simulink model "xhand_sphere_tube_r2021b"  (R2021b)
settings: Solver=VariableStepAuto  StartTime=0.0  StopTime=20  RelTol=1e-3
InitFcn:
  | radium=0.045
undefined symbols (not defined in the file): X, Y, Z
libraries: sm_lib x120, nesl_utility x26, Contact_Forces_Lib x21
(part 2 of 4)

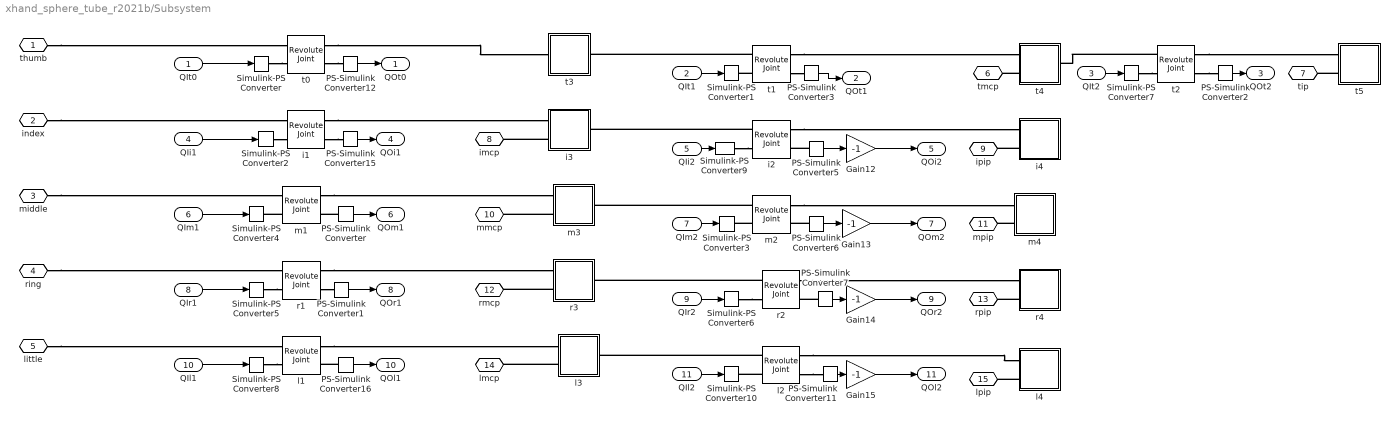
== system xhand_sphere_tube_r2021b/Subsystem ==
  QIt0 : Inport
  QIt1 : Inport  Port=2
  QIt2 : Inport  Port=3
  QIi1 : Inport  Port=4
  QIi2 : Inport  Port=5
  QIm1 : Inport  Port=6
  QIm2 : Inport  Port=7
  QIr1 : Inport  Port=8
  QIr2 : Inport  Port=9
  QIl1 : Inport  Port=10
  QIl2 : Inport  Port=11
  Gain{12..15} (4 alike) : Gain  Gain=-1
  PS-Simulink Converter{,1..3,5..7,11..12,15..16} (11 alike) : nesl_utility/PS-Simulink Converter  PhysicalDomain=network_engine_domain  SubClassName=ps_output  LeftPortType=input  RightPortType=output  PseudoPeriodic=off  Frequencies=[]  Unit=inherit  AffineConversion=off
      settings: SourceProductBaseCode=PW,SS
  Simulink-PS Converter{,1..10} (11 alike) : nesl_utility/Simulink-PS Converter  PhysicalDomain=network_engine_domain  SubClassName=ps_input  LeftPortType=input  RightPortType=output  PseudoPeriodic=off  Frequencies=[]  NoiseDistribution=none  NoiseParameters=[]  Unit=1  AffineConversion=off  FilteringAndDerivatives=filter  SimscapeFilterOrder=2  InputFilterTimeConstant=0.001  UdotUserProvided=0
      settings: SourceProductBaseCode=PW,SS
  i1 : sm_lib/Joints/Revolute Joint  JointMode=Normal  SenseConstraintForce=off  SenseConstraintForceX=off  SenseConstraintForceY=off  SenseConstraintForceZ=off  SenseConstraintTorque=off  SenseConstraintTorqueX=off  SenseConstraintTorqueY=off  SenseConstraintTorqueZ=off  SenseTotalForce=off  SenseTotalForceX=off  SenseTotalForceY=off  SenseTotalForceZ=off  SenseTotalTorque=off  SenseTotalTorqueX=off  SenseTotalTorqueY=off  SenseTotalTorqueZ=off  CompositeWrenchDir=FollowerOnBase  CompositeWrenchFrame=BaseFrame  EquilibriumPosition=0  EquilibriumPositionUnits=deg  SpringStiffness=0  SpringStiffnessUnits=N*m/deg  DampingCoefficient=0  DampingCoefficientUnits=m^2*kg/s/rad  TorqueActuationMode=ComputedTorque  MotionActuationMode=InputMotion  SensePosition=on  SenseVelocity=off  SenseAcceleration=off  SenseTorqueForce=off  SenseLowerLimitTorqueForce=off  SenseUpperLimitTorqueForce=off  LowerLimitSpecify=on  LowerLimitBound=-3.14  LowerLimitBoundUnits=rad  LowerLimitStiffness=1e4  LowerLimitStiffnessUnits=N*m/deg  LowerLimitDamping=10  LowerLimitDampingUnits=N*m/(deg/s)  LowerLimitTransitionRegionWidth=0.1  LowerLimitTransitionRegionWidthUnits=deg  UpperLimitSpecify=on  UpperLimitBound=3.14  UpperLimitBoundUnits=rad  UpperLimitStiffness=1e4  UpperLimitStiffnessUnits=N*m/deg  UpperLimitDamping=10  UpperLimitDampingUnits=N*m/(deg/s)  UpperLimitTransitionRegionWidth=0.1  UpperLimitTransitionRegionWidthUnits=deg  PositionTargetSpecify=off  PositionTargetPriority=High  PositionTargetValue=0  PositionTargetValueUnits=deg  VelocityTargetSpecify=off  VelocityTargetPriority=High  VelocityTargetValue=0  VelocityTargetValueUnits=deg/s
  i2 : sm_lib/Joints/Revolute Joint  JointMode=Normal  SenseConstraintForce=off  SenseConstraintForceX=off  SenseConstraintForceY=off  SenseConstraintForceZ=off  SenseConstraintTorque=off  SenseConstraintTorqueX=off  SenseConstraintTorqueY=off  SenseConstraintTorqueZ=off  SenseTotalForce=off  SenseTotalForceX=off  SenseTotalForceY=off  SenseTotalForceZ=off  SenseTotalTorque=off  SenseTotalTorqueX=off  SenseTotalTorqueY=off  SenseTotalTorqueZ=off  CompositeWrenchDir=FollowerOnBase  CompositeWrenchFrame=BaseFrame  EquilibriumPosition=0  EquilibriumPositionUnits=deg  SpringStiffness=0  SpringStiffnessUnits=N*m/deg  DampingCoefficient=0  DampingCoefficientUnits=m^2*kg/s/rad  TorqueActuationMode=ComputedTorque  MotionActuationMode=InputMotion  SensePosition=on  SenseVelocity=off  SenseAcceleration=off  SenseTorqueForce=off  SenseLowerLimitTorqueForce=off  SenseUpperLimitTorqueForce=off  LowerLimitSpecify=on  LowerLimitBound=-3.14  LowerLimitBoundUnits=rad  LowerLimitStiffness=1e4  LowerLimitStiffnessUnits=N*m/deg  LowerLimitDamping=10  LowerLimitDampingUnits=N*m/(deg/s)  LowerLimitTransitionRegionWidth=0.1  LowerLimitTransitionRegionWidthUnits=deg  UpperLimitSpecify=on  UpperLimitBound=3.14  UpperLimitBoundUnits=rad  UpperLimitStiffness=1e4  UpperLimitStiffnessUnits=N*m/deg  UpperLimitDamping=10  UpperLimitDampingUnits=N*m/(deg/s)  UpperLimitTransitionRegionWidth=0.1  UpperLimitTransitionRegionWidthUnits=deg  PositionTargetSpecify=off  PositionTargetPriority=High  PositionTargetValue=0  PositionTargetValueUnits=deg  VelocityTargetSpecify=off  VelocityTargetPriority=High  VelocityTargetValue=0  VelocityTargetValueUnits=deg/s
  i3 : Subsystem
  i4 : Subsystem
  l1 : sm_lib/Joints/Revolute Joint  JointMode=Normal  SenseConstraintForce=off  SenseConstraintForceX=off  SenseConstraintForceY=off  SenseConstraintForceZ=off  SenseConstraintTorque=off  SenseConstraintTorqueX=off  SenseConstraintTorqueY=off  SenseConstraintTorqueZ=off  SenseTotalForce=off  SenseTotalForceX=off  SenseTotalForceY=off  SenseTotalForceZ=off  SenseTotalTorque=off  SenseTotalTorqueX=off  SenseTotalTorqueY=off  SenseTotalTorqueZ=off  CompositeWrenchDir=FollowerOnBase  CompositeWrenchFrame=BaseFrame  EquilibriumPosition=0  EquilibriumPositionUnits=deg  SpringStiffness=0  SpringStiffnessUnits=N*m/deg  DampingCoefficient=0  DampingCoefficientUnits=m^2*kg/s/rad  TorqueActuationMode=ComputedTorque  MotionActuationMode=InputMotion  SensePosition=on  SenseVelocity=off  SenseAcceleration=off  SenseTorqueForce=off  SenseLowerLimitTorqueForce=off  SenseUpperLimitTorqueForce=off  LowerLimitSpecify=on  LowerLimitBound=-3.14  LowerLimitBoundUnits=rad  LowerLimitStiffness=1e4  LowerLimitStiffnessUnits=N*m/deg  LowerLimitDamping=10  LowerLimitDampingUnits=N*m/(deg/s)  LowerLimitTransitionRegionWidth=0.1  LowerLimitTransitionRegionWidthUnits=deg  UpperLimitSpecify=on  UpperLimitBound=3.14  UpperLimitBoundUnits=rad  UpperLimitStiffness=1e4  UpperLimitStiffnessUnits=N*m/deg  UpperLimitDamping=10  UpperLimitDampingUnits=N*m/(deg/s)  UpperLimitTransitionRegionWidth=0.1  UpperLimitTransitionRegionWidthUnits=deg  PositionTargetSpecify=off  PositionTargetPriority=High  PositionTargetValue=0  PositionTargetValueUnits=deg  VelocityTargetSpecify=off  VelocityTargetPriority=High  VelocityTargetValue=0  VelocityTargetValueUnits=deg/s
  l2 : sm_lib/Joints/Revolute Joint  JointMode=Normal  SenseConstraintForce=off  SenseConstraintForceX=off  SenseConstraintForceY=off  SenseConstraintForceZ=off  SenseConstraintTorque=off  SenseConstraintTorqueX=off  SenseConstraintTorqueY=off  SenseConstraintTorqueZ=off  SenseTotalForce=off  SenseTotalForceX=off  SenseTotalForceY=off  SenseTotalForceZ=off  SenseTotalTorque=off  SenseTotalTorqueX=off  SenseTotalTorqueY=off  SenseTotalTorqueZ=off  CompositeWrenchDir=FollowerOnBase  CompositeWrenchFrame=BaseFrame  EquilibriumPosition=0  EquilibriumPositionUnits=deg  SpringStiffness=0  SpringStiffnessUnits=N*m/deg  DampingCoefficient=0  DampingCoefficientUnits=m^2*kg/s/rad  TorqueActuationMode=ComputedTorque  MotionActuationMode=InputMotion  SensePosition=on  SenseVelocity=off  SenseAcceleration=off  SenseTorqueForce=off  SenseLowerLimitTorqueForce=off  SenseUpperLimitTorqueForce=off  LowerLimitSpecify=on  LowerLimitBound=-3.14  LowerLimitBoundUnits=rad  LowerLimitStiffness=1e4  LowerLimitStiffnessUnits=N*m/deg  LowerLimitDamping=10  LowerLimitDampingUnits=N*m/(deg/s)  LowerLimitTransitionRegionWidth=0.1  LowerLimitTransitionRegionWidthUnits=deg  UpperLimitSpecify=on  UpperLimitBound=3.14  UpperLimitBoundUnits=rad  UpperLimitStiffness=1e4  UpperLimitStiffnessUnits=N*m/deg  UpperLimitDamping=10  UpperLimitDampingUnits=N*m/(deg/s)  UpperLimitTransitionRegionWidth=0.1  UpperLimitTransitionRegionWidthUnits=deg  PositionTargetSpecify=off  PositionTargetPriority=High  PositionTargetValue=0  PositionTargetValueUnits=deg  VelocityTargetSpecify=off  VelocityTargetPriority=High  VelocityTargetValue=0  VelocityTargetValueUnits=deg/s
  l3 : Subsystem
  l4 : Subsystem
  m1 : sm_lib/Joints/Revolute Joint  JointMode=Normal  SenseConstraintForce=off  SenseConstraintForceX=off  SenseConstraintForceY=off  SenseConstraintForceZ=off  SenseConstraintTorque=off  SenseConstraintTorqueX=off  SenseConstraintTorqueY=off  SenseConstraintTorqueZ=off  SenseTotalForce=off  SenseTotalForceX=off  SenseTotalForceY=off  SenseTotalForceZ=off  SenseTotalTorque=off  SenseTotalTorqueX=off  SenseTotalTorqueY=off  SenseTotalTorqueZ=off  CompositeWrenchDir=FollowerOnBase  CompositeWrenchFrame=BaseFrame  EquilibriumPosition=0  EquilibriumPositionUnits=deg  SpringStiffness=0  SpringStiffnessUnits=N*m/deg  DampingCoefficient=0.000005  DampingCoefficientUnits=m^2*kg/s/rad  TorqueActuationMode=ComputedTorque  MotionActuationMode=InputMotion  SensePosition=on  SenseVelocity=off  SenseAcceleration=off  SenseTorqueForce=off  SenseLowerLimitTorqueForce=off  SenseUpperLimitTorqueForce=off  LowerLimitSpecify=on  LowerLimitBound=-3.14  LowerLimitBoundUnits=rad  LowerLimitStiffness=1e4  LowerLimitStiffnessUnits=N*m/deg  LowerLimitDamping=10  LowerLimitDampingUnits=N*m/(deg/s)  LowerLimitTransitionRegionWidth=0.1  LowerLimitTransitionRegionWidthUnits=deg  UpperLimitSpecify=on  UpperLimitBound=3.14  UpperLimitBoundUnits=rad  UpperLimitStiffness=1e4  UpperLimitStiffnessUnits=N*m/deg  UpperLimitDamping=10  UpperLimitDampingUnits=N*m/(deg/s)  UpperLimitTransitionRegionWidth=0.1  UpperLimitTransitionRegionWidthUnits=deg  PositionTargetSpecify=off  PositionTargetPriority=High  PositionTargetValue=0  PositionTargetValueUnits=deg  VelocityTargetSpecify=off  VelocityTargetPriority=High  VelocityTargetValue=0  VelocityTargetValueUnits=deg/s
  m2 : sm_lib/Joints/Revolute Joint  JointMode=Normal  SenseConstraintForce=off  SenseConstraintForceX=off  SenseConstraintForceY=off  SenseConstraintForceZ=off  SenseConstraintTorque=off  SenseConstraintTorqueX=off  SenseConstraintTorqueY=off  SenseConstraintTorqueZ=off  SenseTotalForce=off  SenseTotalForceX=off  SenseTotalForceY=off  SenseTotalForceZ=off  SenseTotalTorque=off  SenseTotalTorqueX=off  SenseTotalTorqueY=off  SenseTotalTorqueZ=off  CompositeWrenchDir=FollowerOnBase  CompositeWrenchFrame=BaseFrame  EquilibriumPosition=0  EquilibriumPositionUnits=deg  SpringStiffness=0  SpringStiffnessUnits=N*m/deg  DampingCoefficient=0  DampingCoefficientUnits=m^2*kg/s/rad  TorqueActuationMode=ComputedTorque  MotionActuationMode=InputMotion  SensePosition=on  SenseVelocity=off  SenseAcceleration=off  SenseTorqueForce=off  SenseLowerLimitTorqueForce=off  SenseUpperLimitTorqueForce=off  LowerLimitSpecify=on  LowerLimitBound=-3.14  LowerLimitBoundUnits=rad  LowerLimitStiffness=1e4  LowerLimitStiffnessUnits=N*m/deg  LowerLimitDamping=10  LowerLimitDampingUnits=N*m/(deg/s)  LowerLimitTransitionRegionWidth=0.1  LowerLimitTransitionRegionWidthUnits=deg  UpperLimitSpecify=on  UpperLimitBound=3.14  UpperLimitBoundUnits=rad  UpperLimitStiffness=1e4  UpperLimitStiffnessUnits=N*m/deg  UpperLimitDamping=10  UpperLimitDampingUnits=N*m/(deg/s)  UpperLimitTransitionRegionWidth=0.1  UpperLimitTransitionRegionWidthUnits=deg  PositionTargetSpecify=off  PositionTargetPriority=High  PositionTargetValue=0  PositionTargetValueUnits=deg  VelocityTargetSpecify=off  VelocityTargetPriority=High  VelocityTargetValue=0  VelocityTargetValueUnits=deg/s
  m3 : Subsystem
  m4 : Subsystem
  r1 : sm_lib/Joints/Revolute Joint  JointMode=Normal  SenseConstraintForce=off  SenseConstraintForceX=off  SenseConstraintForceY=off  SenseConstraintForceZ=off  SenseConstraintTorque=off  SenseConstraintTorqueX=off  SenseConstraintTorqueY=off  SenseConstraintTorqueZ=off  SenseTotalForce=off  SenseTotalForceX=off  SenseTotalForceY=off  SenseTotalForceZ=off  SenseTotalTorque=off  SenseTotalTorqueX=off  SenseTotalTorqueY=off  SenseTotalTorqueZ=off  CompositeWrenchDir=FollowerOnBase  CompositeWrenchFrame=BaseFrame  EquilibriumPosition=0  EquilibriumPositionUnits=deg  SpringStiffness=0  SpringStiffnessUnits=N*m/deg  DampingCoefficient=0.00005  DampingCoefficientUnits=m^2*kg/s/rad  TorqueActuationMode=ComputedTorque  MotionActuationMode=InputMotion  SensePosition=on  SenseVelocity=off  SenseAcceleration=off  SenseTorqueForce=off  SenseLowerLimitTorqueForce=off  SenseUpperLimitTorqueForce=off  LowerLimitSpecify=on  LowerLimitBound=-3.14  LowerLimitBoundUnits=rad  LowerLimitStiffness=1e4  LowerLimitStiffnessUnits=N*m/deg  LowerLimitDamping=10  LowerLimitDampingUnits=N*m/(deg/s)  LowerLimitTransitionRegionWidth=0.1  LowerLimitTransitionRegionWidthUnits=deg  UpperLimitSpecify=on  UpperLimitBound=3.14  UpperLimitBoundUnits=rad  UpperLimitStiffness=1e4  UpperLimitStiffnessUnits=N*m/deg  UpperLimitDamping=10  UpperLimitDampingUnits=N*m/(deg/s)  UpperLimitTransitionRegionWidth=0.1  UpperLimitTransitionRegionWidthUnits=deg  PositionTargetSpecify=off  PositionTargetPriority=High  PositionTargetValue=0  PositionTargetValueUnits=deg  VelocityTargetSpecify=off  VelocityTargetPriority=High  VelocityTargetValue=0  VelocityTargetValueUnits=deg/s
  r2 : sm_lib/Joints/Revolute Joint  JointMode=Normal  SenseConstraintForce=off  SenseConstraintForceX=off  SenseConstraintForceY=off  SenseConstraintForceZ=off  SenseConstraintTorque=off  SenseConstraintTorqueX=off  SenseConstraintTorqueY=off  SenseConstraintTorqueZ=off  SenseTotalForce=off  SenseTotalForceX=off  SenseTotalForceY=off  SenseTotalForceZ=off  SenseTotalTorque=off  SenseTotalTorqueX=off  SenseTotalTorqueY=off  SenseTotalTorqueZ=off  CompositeWrenchDir=FollowerOnBase  CompositeWrenchFrame=BaseFrame  EquilibriumPosition=0  EquilibriumPositionUnits=deg  SpringStiffness=0  SpringStiffnessUnits=N*m/deg  DampingCoefficient=0  DampingCoefficientUnits=m^2*kg/s/rad  TorqueActuationMode=ComputedTorque  MotionActuationMode=InputMotion  SensePosition=on  SenseVelocity=off  SenseAcceleration=off  SenseTorqueForce=off  SenseLowerLimitTorqueForce=off  SenseUpperLimitTorqueForce=off  LowerLimitSpecify=on  LowerLimitBound=-3.14  LowerLimitBoundUnits=rad  LowerLimitStiffness=1e4  LowerLimitStiffnessUnits=N*m/deg  LowerLimitDamping=10  LowerLimitDampingUnits=N*m/(deg/s)  LowerLimitTransitionRegionWidth=0.1  LowerLimitTransitionRegionWidthUnits=deg  UpperLimitSpecify=on  UpperLimitBound=3.14  UpperLimitBoundUnits=rad  UpperLimitStiffness=1e4  UpperLimitStiffnessUnits=N*m/deg  UpperLimitDamping=10  UpperLimitDampingUnits=N*m/(deg/s)  UpperLimitTransitionRegionWidth=0.1  UpperLimitTransitionRegionWidthUnits=deg  PositionTargetSpecify=off  PositionTargetPriority=High  PositionTargetValue=0  PositionTargetValueUnits=deg  VelocityTargetSpecify=off  VelocityTargetPriority=High  VelocityTargetValue=0  VelocityTargetValueUnits=deg/s
  r3 : Subsystem
  r4 : Subsystem
  t0 : sm_lib/Joints/Revolute Joint  JointMode=Normal  SenseConstraintForce=off  SenseConstraintForceX=off  SenseConstraintForceY=off  SenseConstraintForceZ=off  SenseConstraintTorque=off  SenseConstraintTorqueX=off  SenseConstraintTorqueY=off  SenseConstraintTorqueZ=off  SenseTotalForce=off  SenseTotalForceX=off  SenseTotalForceY=off  SenseTotalForceZ=off  SenseTotalTorque=off  SenseTotalTorqueX=off  SenseTotalTorqueY=off  SenseTotalTorqueZ=off  CompositeWrenchDir=FollowerOnBase  CompositeWrenchFrame=BaseFrame  EquilibriumPosition=0  EquilibriumPositionUnits=deg  SpringStiffness=0  SpringStiffnessUnits=N*m/deg  DampingCoefficient=0  DampingCoefficientUnits=m^2*kg/s/rad  TorqueActuationMode=ComputedTorque  MotionActuationMode=InputMotion  SensePosition=on  SenseVelocity=off  SenseAcceleration=off  SenseTorqueForce=off  SenseLowerLimitTorqueForce=off  SenseUpperLimitTorqueForce=off  LowerLimitSpecify=on  LowerLimitBound=-3.14  LowerLimitBoundUnits=rad  LowerLimitStiffness=1e4  LowerLimitStiffnessUnits=N*m/deg  LowerLimitDamping=10  LowerLimitDampingUnits=N*m/(deg/s)  LowerLimitTransitionRegionWidth=0.1  LowerLimitTransitionRegionWidthUnits=deg  UpperLimitSpecify=on  UpperLimitBound=3.14  UpperLimitBoundUnits=rad  UpperLimitStiffness=1e4  UpperLimitStiffnessUnits=N*m/deg  UpperLimitDamping=10  UpperLimitDampingUnits=N*m/(deg/s)  UpperLimitTransitionRegionWidth=0.1  UpperLimitTransitionRegionWidthUnits=deg  PositionTargetSpecify=off  PositionTargetPriority=High  PositionTargetValue=0  PositionTargetValueUnits=deg  VelocityTargetSpecify=off  VelocityTargetPriority=High  VelocityTargetValue=0  VelocityTargetValueUnits=deg/s
  t1 : sm_lib/Joints/Revolute Joint  JointMode=Normal  SenseConstraintForce=off  SenseConstraintForceX=off  SenseConstraintForceY=off  SenseConstraintForceZ=off  SenseConstraintTorque=off  SenseConstraintTorqueX=off  SenseConstraintTorqueY=off  SenseConstraintTorqueZ=off  SenseTotalForce=off  SenseTotalForceX=off  SenseTotalForceY=off  SenseTotalForceZ=off  SenseTotalTorque=off  SenseTotalTorqueX=off  SenseTotalTorqueY=off  SenseTotalTorqueZ=off  CompositeWrenchDir=FollowerOnBase  CompositeWrenchFrame=BaseFrame  EquilibriumPosition=0  EquilibriumPositionUnits=deg  SpringStiffness=0  SpringStiffnessUnits=N*m/deg  DampingCoefficient=0  DampingCoefficientUnits=m^2*kg/s/rad  TorqueActuationMode=ComputedTorque  MotionActuationMode=InputMotion  SensePosition=on  SenseVelocity=off  SenseAcceleration=off  SenseTorqueForce=off  SenseLowerLimitTorqueForce=off  SenseUpperLimitTorqueForce=off  LowerLimitSpecify=on  LowerLimitBound=-3.14  LowerLimitBoundUnits=rad  LowerLimitStiffness=1e4  LowerLimitStiffnessUnits=N*m/deg  LowerLimitDamping=10  LowerLimitDampingUnits=N*m/(deg/s)  LowerLimitTransitionRegionWidth=0.1  LowerLimitTransitionRegionWidthUnits=deg  UpperLimitSpecify=on  UpperLimitBound=3.14  UpperLimitBoundUnits=rad  UpperLimitStiffness=1e4  UpperLimitStiffnessUnits=N*m/deg  UpperLimitDamping=10  UpperLimitDampingUnits=N*m/(deg/s)  UpperLimitTransitionRegionWidth=0.1  UpperLimitTransitionRegionWidthUnits=deg  PositionTargetSpecify=off  PositionTargetPriority=High  PositionTargetValue=0  PositionTargetValueUnits=deg  VelocityTargetSpecify=off  VelocityTargetPriority=High  VelocityTargetValue=0  VelocityTargetValueUnits=deg/s
  t2 : sm_lib/Joints/Revolute Joint  JointMode=Normal  SenseConstraintForce=off  SenseConstraintForceX=off  SenseConstraintForceY=off  SenseConstraintForceZ=off  SenseConstraintTorque=off  SenseConstraintTorqueX=off  SenseConstraintTorqueY=off  SenseConstraintTorqueZ=off  SenseTotalForce=off  SenseTotalForceX=off  SenseTotalForceY=off  SenseTotalForceZ=off  SenseTotalTorque=off  SenseTotalTorqueX=off  SenseTotalTorqueY=off  SenseTotalTorqueZ=off  CompositeWrenchDir=FollowerOnBase  CompositeWrenchFrame=BaseFrame  EquilibriumPosition=0  EquilibriumPositionUnits=deg  SpringStiffness=0  SpringStiffnessUnits=N*m/deg  DampingCoefficient=0  DampingCoefficientUnits=m^2*kg/s/rad  TorqueActuationMode=ComputedTorque  MotionActuationMode=InputMotion  SensePosition=on  SenseVelocity=off  SenseAcceleration=off  SenseTorqueForce=off  SenseLowerLimitTorqueForce=off  SenseUpperLimitTorqueForce=off  LowerLimitSpecify=on  LowerLimitBound=-3.14  LowerLimitBoundUnits=rad  LowerLimitStiffness=1e4  LowerLimitStiffnessUnits=N*m/deg  LowerLimitDamping=10  LowerLimitDampingUnits=N*m/(deg/s)  LowerLimitTransitionRegionWidth=0.1  LowerLimitTransitionRegionWidthUnits=deg  UpperLimitSpecify=on  UpperLimitBound=3.14  UpperLimitBoundUnits=rad  UpperLimitStiffness=1e4  UpperLimitStiffnessUnits=N*m/deg  UpperLimitDamping=10  UpperLimitDampingUnits=N*m/(deg/s)  UpperLimitTransitionRegionWidth=0.1  UpperLimitTransitionRegionWidthUnits=deg  PositionTargetSpecify=off  PositionTargetPriority=High  PositionTargetValue=0  PositionTargetValueUnits=deg  VelocityTargetSpecify=off  VelocityTargetPriority=High  VelocityTargetValue=0  VelocityTargetValueUnits=deg/s
  t3 : Subsystem
  t4 : Subsystem
  t5 : Subsystem
  thumb : PMIOPort  Side=Left
  index : PMIOPort  Port=2  Side=Left
  middle : PMIOPort  Port=3  Side=Left
  ring : PMIOPort  Port=4  Side=Left
  little : PMIOPort  Port=5  Side=Left
  tmcp : PMIOPort  Port=6  Side=Left
  tip : PMIOPort  Port=7  Side=Left
  imcp : PMIOPort  Port=8  Side=Left
  ipip : PMIOPort  Port=9  Side=Left
  mmcp : PMIOPort  Port=10  Side=Left
  mpip : PMIOPort  Port=11  Side=Left
  rmcp : PMIOPort  Port=12  Side=Left
  rpip : PMIOPort  Port=13  Side=Left
  lmcp : PMIOPort  Port=14  Side=Left
  lpip : PMIOPort  Port=15  Side=Left
  QOt0 : Outport
  QOt1 : Outport  Port=2
  QOt2 : Outport  Port=3
  QOi1 : Outport  Port=4
  QOi2 : Outport  Port=5
  QOm1 : Outport  Port=6
  QOm2 : Outport  Port=7
  QOr1 : Outport  Port=8
  QOr2 : Outport  Port=9
  QOl1 : Outport  Port=10
  QOl2 : Outport  Port=11
  wires:
  Gain13/1 -> QOm2/1
  PS-Simulink Converter5/1 -> Gain12/1
  QIm2/1 -> Simulink-PS Converter3/1
  QIt1/1 -> Simulink-PS Converter1/1
  PS-Simulink Converter11/1 -> Gain15/1
  PS-Simulink Converter6/1 -> Gain13/1
  PS-Simulink Converter2/1 -> QOt2/1
  Gain14/1 -> QOr2/1
  PS-Simulink Converter7/1 -> Gain14/1
  Gain12/1 -> QOi2/1
  PS-Simulink Converter12/1 -> QOt0/1
  QIr1/1 -> Simulink-PS Converter5/1
  PS-Simulink Converter/1 -> QOm1/1
  PS-Simulink Converter1/1 -> QOr1/1
  Gain15/1 -> QOl2/1
  PS-Simulink Converter16/1 -> QOl1/1
  PS-Simulink Converter3/1 -> QOt1/1
  QIi2/1 -> Simulink-PS Converter9/1
  QIr2/1 -> Simulink-PS Converter6/1
  QIl2/1 -> Simulink-PS Converter10/1
  QIi1/1 -> Simulink-PS Converter2/1
  QIt0/1 -> Simulink-PS Converter/1
  QIl1/1 -> Simulink-PS Converter8/1
  QIm1/1 -> Simulink-PS Converter4/1
  QIt2/1 -> Simulink-PS Converter7/1
  PS-Simulink Converter15/1 -> QOi1/1
  connections:
  Simulink-PS Converter9/RConn1 -- i2/LConn2
  m1/RConn1 -- m3/LConn1
  Simulink-PS Converter2/RConn1 -- i1/LConn2
  t1/LConn2 -- Simulink-PS Converter1/RConn1
  i2/RConn1 -- i4/LConn1
  t2/LConn1 -- t4/RConn1
  l2/LConn2 -- Simulink-PS Converter10/RConn1
  m4/LConn2 -- mpip/RConn1
  m3/LConn2 -- mmcp/RConn1
  Simulink-PS Converter8/RConn1 -- l1/LConn2
  PS-Simulink Converter7/LConn1 -- r2/RConn2
  r2/RConn1 -- r4/LConn1
  i1/RConn1 -- i3/LConn1
  t0/RConn1 -- t3/LConn1
  i2/LConn1 -- i3/RConn1
  t2/RConn1 -- t5/LConn1
  t1/RConn1 -- t4/LConn1
  t0/RConn2 -- PS-Simulink Converter12/LConn1
  l1/RConn1 -- l3/LConn1
  t1/LConn1 -- t3/RConn1
  t1/RConn2 -- PS-Simulink Converter3/LConn1
  m2/LConn1 -- m3/RConn1
  m2/LConn2 -- Simulink-PS Converter3/RConn1
  Simulink-PS Converter5/RConn1 -- r1/LConn2
  l2/RConn2 -- PS-Simulink Converter11/LConn1
  i4/LConn2 -- ipip/RConn1
  index/RConn1 -- i1/LConn1
  PS-Simulink Converter6/LConn1 -- m2/RConn2
  Simulink-PS Converter6/RConn1 -- r2/LConn2
  i1/RConn2 -- PS-Simulink Converter15/LConn1
  l3/LConn2 -- lmcp/RConn1
  r1/RConn1 -- r3/LConn1
  thumb/RConn1 -- t0/LConn1
  PS-Simulink Converter/LConn1 -- m1/RConn2
  l2/RConn1 -- l4/LConn1
  little/RConn1 -- l1/LConn1
  middle/RConn1 -- m1/LConn1
  r2/LConn1 -- r3/RConn1
  PS-Simulink Converter16/LConn1 -- l1/RConn2
  Simulink-PS Converter7/RConn1 -- t2/LConn2
  r1/RConn2 -- PS-Simulink Converter1/LConn1
  PS-Simulink Converter5/LConn1 -- i2/RConn2
  l4/LConn2 -- lpip/RConn1
  t2/RConn2 -- PS-Simulink Converter2/LConn1
  l2/LConn1 -- l3/RConn1
  r3/LConn2 -- rmcp/RConn1
  m2/RConn1 -- m4/LConn1
  Simulink-PS Converter/RConn1 -- t0/LConn2
  ring/RConn1 -- r1/LConn1
  m1/LConn2 -- Simulink-PS Converter4/RConn1
  r4/LConn2 -- rpip/RConn1
  t4/LConn2 -- tmcp/RConn1
  i3/LConn2 -- imcp/RConn1
  t5/LConn2 -- tip/RConn1

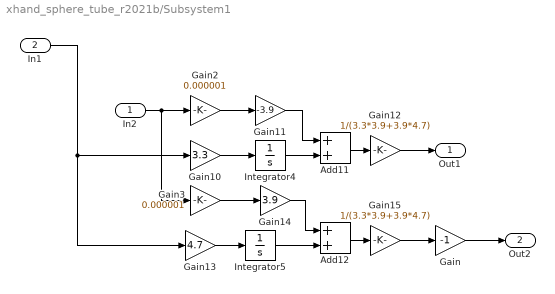
== system xhand_sphere_tube_r2021b/Subsystem1 ==
  In2 : Inport
  In1 : Inport  Port=2
  Add11 : Sum
  Add12 : Sum
  Gain : Gain  Gain=-1
  Gain10 : Gain  Gain=3.3
  Gain11 : Gain  Gain=-3.9
  Gain12 : Gain  Gain=1/(3.3*3.9+3.9*4.7)
  Gain13 : Gain  Gain=4.7
  Gain14 : Gain  Gain=3.9
  Gain15 : Gain  Gain=1/(3.3*3.9+3.9*4.7)
  Gain2 : Gain  Gain=0.000001
  Gain3 : Gain  Gain=0.000001
  Integrator4 : Integrator
  Integrator5 : Integrator
  Out1 : Outport
  Out2 : Outport  Port=2
  wires:
  Gain13/1 -> Integrator5/1
  Add12/1 -> Gain15/1
  In2/1 -> Gain2/1, Gain3/1
  Integrator5/1 -> Add12/2
  In1/1 -> Gain13/1, Gain10/1
  Gain14/1 -> Add12/1
  Integrator4/1 -> Add11/2
  Gain10/1 -> Integrator4/1
  Gain12/1 -> Out1/1
  Gain15/1 -> Gain/1
  Gain11/1 -> Add11/1
  Gain2/1 -> Gain11/1
  Add11/1 -> Gain12/1
  Gain3/1 -> Gain14/1
  Gain/1 -> Out2/1

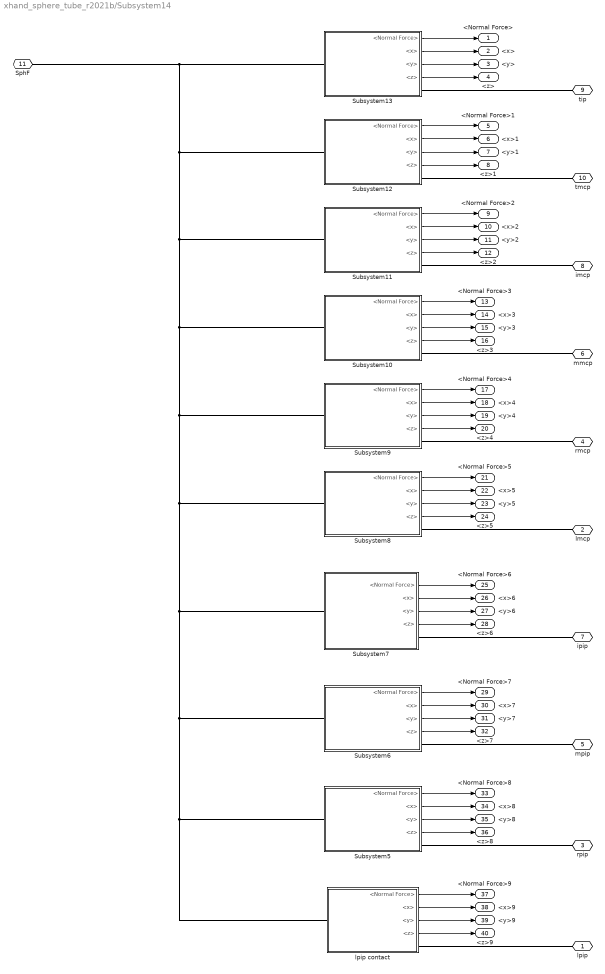
== system xhand_sphere_tube_r2021b/Subsystem14 ==
  Subsystem10 : Subsystem
  Subsystem11 : Subsystem
  Subsystem12 : Subsystem
  Subsystem13 : Subsystem
  Subsystem5 : Subsystem
  Subsystem6 : Subsystem
  Subsystem7 : Subsystem
  Subsystem8 : Subsystem
  Subsystem9 : Subsystem
  lpip contact : Subsystem
  lpip : PMIOPort  Side=Left
  lmcp : PMIOPort  Port=2  Side=Left
  rpip : PMIOPort  Port=3  Side=Left
  rmcp : PMIOPort  Port=4  Side=Left
  mpip : PMIOPort  Port=5  Side=Left
  mmcp : PMIOPort  Port=6  Side=Left
  ipip : PMIOPort  Port=7  Side=Left
  imcp : PMIOPort  Port=8  Side=Left
  tip : PMIOPort  Port=9  Side=Left
  tmcp : PMIOPort  Port=10  Side=Left
  SphF : PMIOPort  Port=11  Side=Left
  <Normal Force> : Outport
  <x> : Outport  Port=2
  <y> : Outport  Port=3
  <z> : Outport  Port=4
  <Normal Force>1 : Outport  Port=5
  <x>1 : Outport  Port=6
  <y>1 : Outport  Port=7
  <z>1 : Outport  Port=8
  <Normal Force>2 : Outport  Port=9
  <x>2 : Outport  Port=10
  <y>2 : Outport  Port=11
  <z>2 : Outport  Port=12
  <Normal Force>3 : Outport  Port=13
  <x>3 : Outport  Port=14
  <y>3 : Outport  Port=15
  <z>3 : Outport  Port=16
  <Normal Force>4 : Outport  Port=17
  <x>4 : Outport  Port=18
  <y>4 : Outport  Port=19
  <z>4 : Outport  Port=20
  <Normal Force>5 : Outport  Port=21
  <x>5 : Outport  Port=22
  <y>5 : Outport  Port=23
  <z>5 : Outport  Port=24
  <Normal Force>6 : Outport  Port=25
  <x>6 : Outport  Port=26
  <y>6 : Outport  Port=27
  <z>6 : Outport  Port=28
  <Normal Force>7 : Outport  Port=29
  <x>7 : Outport  Port=30
  <y>7 : Outport  Port=31
  <z>7 : Outport  Port=32
  <Normal Force>8 : Outport  Port=33
  <x>8 : Outport  Port=34
  <y>8 : Outport  Port=35
  <z>8 : Outport  Port=36
  <Normal Force>9 : Outport  Port=37
  <x>9 : Outport  Port=38
  <y>9 : Outport  Port=39
  <z>9 : Outport  Port=40
  wires:
  Subsystem6/2(<x>) -> <x>7/1
  Subsystem10/4(<z>) -> <z>3/1
  lpip contact/4(<z>) -> <z>9/1
  Subsystem8/4(<z>) -> <z>5/1
  Subsystem6/4(<z>) -> <z>7/1
  Subsystem6/1(<Normal Force>) -> <Normal Force>7/1
  lpip contact/3(<y>) -> <y>9/1
  Subsystem5/3(<y>) -> <y>8/1
  Subsystem7/2(<x>) -> <x>6/1
  Subsystem9/4(<z>) -> <z>4/1
  Subsystem11/1(<Normal Force>) -> <Normal Force>2/1
  Subsystem10/2(<x>) -> <x>3/1
  Subsystem6/3(<y>) -> <y>7/1
  Subsystem9/2(<x>) -> <x>4/1
  Subsystem11/2(<x>) -> <x>2/1
  Subsystem11/3(<y>) -> <y>2/1
  Subsystem7/3(<y>) -> <y>6/1
  Subsystem12/1(<Normal Force>) -> <Normal Force>1/1
  Subsystem9/1(<Normal Force>) -> <Normal Force>4/1
  Subsystem11/4(<z>) -> <z>2/1
  Subsystem5/1(<Normal Force>) -> <Normal Force>8/1
  Subsystem9/3(<y>) -> <y>4/1
  Subsystem10/1(<Normal Force>) -> <Normal Force>3/1
  Subsystem12/3(<y>) -> <y>1/1
  Subsystem12/2(<x>) -> <x>1/1
  Subsystem12/4(<z>) -> <z>1/1
  Subsystem13/3(<y>) -> <y>/1
  Subsystem5/4(<z>) -> <z>8/1
  Subsystem5/2(<x>) -> <x>8/1
  Subsystem13/1(<Normal Force>) -> <Normal Force>/1
  Subsystem7/4(<z>) -> <z>6/1
  Subsystem7/1(<Normal Force>) -> <Normal Force>6/1
  Subsystem8/1(<Normal Force>) -> <Normal Force>5/1
  Subsystem8/2(<x>) -> <x>5/1
  lpip contact/2(<x>) -> <x>9/1
  Subsystem8/3(<y>) -> <y>5/1
  Subsystem10/3(<y>) -> <y>3/1
  lpip contact/1(<Normal Force>) -> <Normal Force>9/1
  Subsystem13/2(<x>) -> <x>/1
  Subsystem13/4(<z>) -> <z>/1
  connections:
  lpip contact/LConn1 -- SphF/RConn1 -- Subsystem13/LConn1 -- Subsystem12/LConn1 -- Subsystem11/LConn1 -- Subsystem10/LConn1 -- Subsystem9/LConn1 -- Subsystem8/LConn1 -- Subsystem7/LConn1 -- Subsystem6/LConn1 -- Subsystem5/LConn1
  Subsystem9/RConn1 -- rmcp/RConn1
  Subsystem6/RConn1 -- mpip/RConn1
  Subsystem11/RConn1 -- imcp/RConn1
  Subsystem10/RConn1 -- mmcp/RConn1
  Subsystem8/RConn1 -- lmcp/RConn1
  Subsystem12/RConn1 -- tmcp/RConn1
  lpip contact/RConn1 -- lpip/RConn1
  Subsystem7/RConn1 -- ipip/RConn1
  rpip/RConn1 -- Subsystem5/RConn1
  Subsystem13/RConn1 -- tip/RConn1

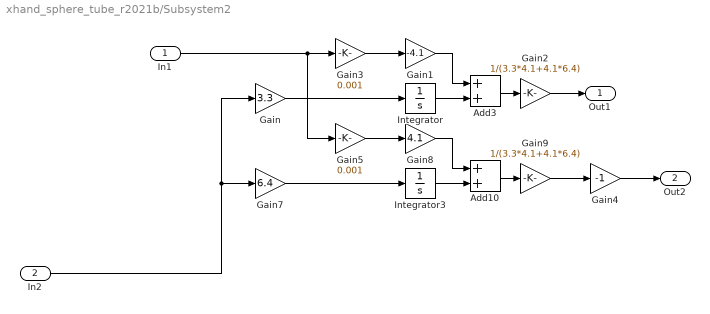
== system xhand_sphere_tube_r2021b/Subsystem2 ==
  In1 : Inport
  In2 : Inport  Port=2
  Add10 : Sum
  Add3 : Sum
  Gain : Gain  Gain=3.3
  Gain1 : Gain  Gain=-4.1
  Gain2 : Gain  Gain=1/(3.3*4.1+4.1*6.4)
  Gain3 : Gain  Gain=0.001
  Gain4 : Gain  Gain=-1
  Gain5 : Gain  Gain=0.001
  Gain7 : Gain  Gain=6.4
  Gain8 : Gain  Gain=4.1
  Gain9 : Gain  Gain=1/(3.3*4.1+4.1*6.4)
  Integrator : Integrator
  Integrator3 : Integrator
  Out1 : Outport
  Out2 : Outport  Port=2
  wires:
  Gain1/1 -> Add3/1
  Gain/1 -> Integrator/1
  Integrator/1 -> Add3/2
  Gain8/1 -> Add10/1
  Integrator3/1 -> Add10/2
  Add3/1 -> Gain2/1
  Gain7/1 -> Integrator3/1
  Add10/1 -> Gain9/1
  In2/1 -> Gain7/1, Gain/1
  In1/1 -> Gain3/1, Gain5/1
  Gain2/1 -> Out1/1
  Gain9/1 -> Gain4/1
  Gain4/1 -> Out2/1
  Gain3/1 -> Gain1/1
  Gain5/1 -> Gain8/1

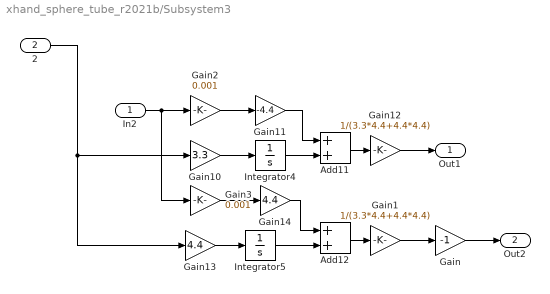
== system xhand_sphere_tube_r2021b/Subsystem3 ==
  In2 : Inport
  2 : Inport  Port=2
  Add11 : Sum
  Add12 : Sum
  Gain : Gain  Gain=-1
  Gain1 : Gain  Gain=1/(3.3*4.4+4.4*4.4)
  Gain10 : Gain  Gain=3.3
  Gain11 : Gain  Gain=-4.4
  Gain12 : Gain  Gain=1/(3.3*4.4+4.4*4.4)
  Gain13 : Gain  Gain=4.4
  Gain14 : Gain  Gain=4.4
  Gain2 : Gain  Gain=0.001
  Gain3 : Gain  Gain=0.001
  Integrator4 : Integrator
  Integrator5 : Integrator
  Out1 : Outport
  Out2 : Outport  Port=2
  wires:
  Gain13/1 -> Integrator5/1
  Add12/1 -> Gain1/1
  In2/1 -> Gain3/1, Gain2/1
  Integrator5/1 -> Add12/2
  2/1 -> Gain13/1, Gain10/1
  Gain14/1 -> Add12/1
  Add11/1 -> Gain12/1
  Integrator4/1 -> Add11/2
  Gain11/1 -> Add11/1
  Gain10/1 -> Integrator4/1
  Gain12/1 -> Out1/1
  Gain1/1 -> Gain/1
  Gain/1 -> Out2/1
  Gain3/1 -> Gain14/1
  Gain2/1 -> Gain11/1

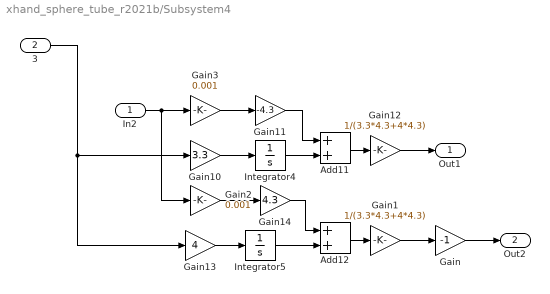
== system xhand_sphere_tube_r2021b/Subsystem4 ==
  In2 : Inport
  3 : Inport  Port=2
  Add11 : Sum
  Add12 : Sum
  Gain : Gain  Gain=-1
  Gain1 : Gain  Gain=1/(3.3*4.3+4*4.3)
  Gain10 : Gain  Gain=3.3
  Gain11 : Gain  Gain=-4.3
  Gain12 : Gain  Gain=1/(3.3*4.3+4*4.3)
  Gain13 : Gain  Gain=4
  Gain14 : Gain  Gain=4.3
  Gain2 : Gain  Gain=0.001
  Gain3 : Gain  Gain=0.001
  Integrator4 : Integrator
  Integrator5 : Integrator
  Out1 : Outport
  Out2 : Outport  Port=2
  wires:
  Gain13/1 -> Integrator5/1
  Add12/1 -> Gain1/1
  In2/1 -> Gain2/1, Gain3/1
  Integrator5/1 -> Add12/2
  3/1 -> Gain13/1, Gain10/1
  Gain14/1 -> Add12/1
  Add11/1 -> Gain12/1
  Integrator4/1 -> Add11/2
  Gain11/1 -> Add11/1
  Gain10/1 -> Integrator4/1
  Gain12/1 -> Out1/1
  Gain1/1 -> Gain/1
  Gain/1 -> Out2/1
  Gain2/1 -> Gain14/1
  Gain3/1 -> Gain11/1

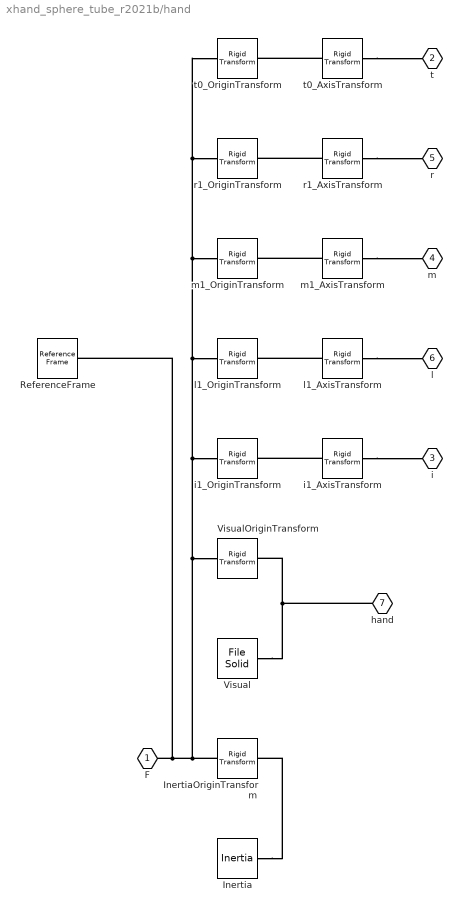
== system xhand_sphere_tube_r2021b/hand ==
  Inertia : sm_lib/Body Elements/Inertia  InertiaType=Custom  Mass=0.076365958538922  MassUnits=kg  CenterOfMass=[0, 0, 0]  CenterOfMassUnits=m  MomentsOfInertia=[5.07424152927554e-05, 5.37071967863805e-05, 0.000100259361691297]  MomentsOfInertiaUnits=kg*m^2  ProductsOfInertia=[2.58578904792979e-07, 1.33961850702105e-07, -2.17892480399571e-07]  ProductsOfInertiaUnits=kg*m^2  GraphicType=None  MarkerShape=Inertia  MarkerSize=20  GraphicVisPropType=SimpleVisualProperties  GraphicDiffuseColor=[0.5 0.5 0.5]  GraphicSpecularColor=[0.5 0.5 0.5 1.0]  GraphicAmbientColor=[0.15 0.15 0.15 1.0]  GraphicEmissiveColor=[0.0 0.0 0.0 1.0]  GraphicShininess=75  GraphicOpacity=1.0
  InertiaOriginTransform : sm_lib/Frames and Transforms/Rigid Transform  TranslationMethod=Cartesian  TranslationStandardOffset=0  TranslationLengthUnit=m  TranslationStandardAxis=+Z  TranslationCartesianOffset=[0.000120501105179326, -0.0331000985791428, -0.0151769506261707]  TranslationROffset=0  TranslationROffsetUnits=m  TranslationZOffset=0  TranslationZOffsetUnits=m  TranslationThetaOffset=0  TranslationThetaOffsetUnits=deg  RotationMethod=RotationSequence  RotationAngleUnits=deg  RotationStandardAxis=+Z  RotationAngle=0.0  RotationArbitraryAxis=[0 0 1]  FollAlignAxisA=+X  BaseAlignAxisA=+Y  FollAlignAxisB=+Y  BaseAlignAxisB=+Z  RotationSequenceAxes=BaseAxes  RotationSequence=XYZ  RotationSequenceAngles=[0, 0, 0]  RotationSequenceAnglesUnits=rad  RotationMatrix=[1 0 0; 0 1 0; 0 0 1]
  ReferenceFrame : sm_lib/Frames and Transforms/Reference Frame
  Visual : sm_lib/Body Elements/File Solid  ExtGeomFileName=xhand/meshes/hand.STL  UnitType=Custom  ExtGeomFileUnits=m  StepReaderType=HEX  ExportConvexHullGeometry=off  InertiaType=Custom  Mass=1000  MassUnits=kg  CenterOfMass=[0, 0, 0]  CenterOfMassUnits=m  MomentsOfInertia=[100,100,100]  MomentsOfInertiaUnits=kg*m^2  ProductsOfInertia=[100, 100, 100]  ProductsOfInertiaUnits=kg*m^2  BasedOnType=DensityFromFile  Density=1000  DensityUnits=kg/m^3  DoExposeReferenceFrame=on  SerializedFrames=<Frames/>  GraphicType=FromGeometry  MarkerShape=Sphere  MarkerSize=10  GraphicVisPropType=SimpleVisualProperties  GraphicDiffuseColor=[1, 1, 1]  GraphicSpecularColor=[0.5 0.5 0.5 1.0]  GraphicAmbientColor=[0.15 0.15 0.15 1.0]  GraphicEmissiveColor=[0.0 0.0 0.0 1.0]  GraphicShininess=75  GraphicOpacity=1
  VisualOriginTransform : sm_lib/Frames and Transforms/Rigid Transform  TranslationMethod=Cartesian  TranslationStandardOffset=0  TranslationLengthUnit=m  TranslationStandardAxis=+Z  TranslationCartesianOffset=[0, 0, 0]  TranslationROffset=0  TranslationROffsetUnits=m  TranslationZOffset=0  TranslationZOffsetUnits=m  TranslationThetaOffset=0  TranslationThetaOffsetUnits=deg  RotationMethod=RotationSequence  RotationAngleUnits=deg  RotationStandardAxis=+Z  RotationAngle=0.0  RotationArbitraryAxis=[0 0 1]  FollAlignAxisA=+X  BaseAlignAxisA=+Y  FollAlignAxisB=+Y  BaseAlignAxisB=+Z  RotationSequenceAxes=BaseAxes  RotationSequence=XYZ  RotationSequenceAngles=[0, 0, 0]  RotationSequenceAnglesUnits=rad  RotationMatrix=[1 0 0; 0 1 0; 0 0 1]
  i1_AxisTransform : sm_lib/Frames and Transforms/Rigid Transform  TranslationMethod=Cartesian  TranslationStandardOffset=0  TranslationLengthUnit=m  TranslationStandardAxis=+Z  TranslationCartesianOffset=[0, 0, 0]  TranslationROffset=0  TranslationROffsetUnits=m  TranslationZOffset=0  TranslationZOffsetUnits=m  TranslationThetaOffset=0  TranslationThetaOffsetUnits=deg  RotationMethod=ArbitraryAxis  RotationAngleUnits=rad  RotationStandardAxis=+Z  RotationAngle=1.570796326794897  RotationArbitraryAxis=[-0, 1, 0]  FollAlignAxisA=+X  BaseAlignAxisA=+Y  FollAlignAxisB=+Y  BaseAlignAxisB=+Z  RotationSequenceAxes=FollowerAxes  RotationSequence=XYX  RotationSequenceAngles=[0 0 0]  RotationSequenceAnglesUnits=deg  RotationMatrix=[1 0 0; 0 1 0; 0 0 1]
  i1_OriginTransform : sm_lib/Frames and Transforms/Rigid Transform  TranslationMethod=Cartesian  TranslationStandardOffset=0  TranslationLengthUnit=m  TranslationStandardAxis=+Z  TranslationCartesianOffset=[0.024667, 0.01527, -0.0165]  TranslationROffset=0  TranslationROffsetUnits=m  TranslationZOffset=0  TranslationZOffsetUnits=m  TranslationThetaOffset=0  TranslationThetaOffsetUnits=deg  RotationMethod=RotationSequence  RotationAngleUnits=deg  RotationStandardAxis=+Z  RotationAngle=0.0  RotationArbitraryAxis=[0 0 1]  FollAlignAxisA=+X  BaseAlignAxisA=+Y  FollAlignAxisB=+Y  BaseAlignAxisB=+Z  RotationSequenceAxes=BaseAxes  RotationSequence=XYZ  RotationSequenceAngles=[0, 0, -0.069813]  RotationSequenceAnglesUnits=rad  RotationMatrix=[1 0 0; 0 1 0; 0 0 1]
  l1_AxisTransform : sm_lib/Frames and Transforms/Rigid Transform  TranslationMethod=Cartesian  TranslationStandardOffset=0  TranslationLengthUnit=m  TranslationStandardAxis=+Z  TranslationCartesianOffset=[0, 0, 0]  TranslationROffset=0  TranslationROffsetUnits=m  TranslationZOffset=0  TranslationZOffsetUnits=m  TranslationThetaOffset=0  TranslationThetaOffsetUnits=deg  RotationMethod=ArbitraryAxis  RotationAngleUnits=rad  RotationStandardAxis=+Z  RotationAngle=1.570796326794897  RotationArbitraryAxis=[-0, 1, 0]  FollAlignAxisA=+X  BaseAlignAxisA=+Y  FollAlignAxisB=+Y  BaseAlignAxisB=+Z  RotationSequenceAxes=FollowerAxes  RotationSequence=XYX  RotationSequenceAngles=[0 0 0]  RotationSequenceAnglesUnits=deg  RotationMatrix=[1 0 0; 0 1 0; 0 0 1]
  l1_OriginTransform : sm_lib/Frames and Transforms/Rigid Transform  TranslationMethod=Cartesian  TranslationStandardOffset=0  TranslationLengthUnit=m  TranslationStandardAxis=+Z  TranslationCartesianOffset=[-0.02725452041389, 0.0106193163170702, -0.0164999999999987]  TranslationROffset=0  TranslationROffsetUnits=m  TranslationZOffset=0  TranslationZOffsetUnits=m  TranslationThetaOffset=0  TranslationThetaOffsetUnits=deg  RotationMethod=RotationSequence  RotationAngleUnits=deg  RotationStandardAxis=+Z  RotationAngle=0.0  RotationArbitraryAxis=[0 0 1]  FollAlignAxisA=+X  BaseAlignAxisA=+Y  FollAlignAxisB=+Y  BaseAlignAxisB=+Z  RotationSequenceAxes=BaseAxes  RotationSequence=XYZ  RotationSequenceAngles=[0, 0, 0.122173047639604]  RotationSequenceAnglesUnits=rad  RotationMatrix=[1 0 0; 0 1 0; 0 0 1]
  m1_AxisTransform : sm_lib/Frames and Transforms/Rigid Transform  TranslationMethod=Cartesian  TranslationStandardOffset=0  TranslationLengthUnit=m  TranslationStandardAxis=+Z  TranslationCartesianOffset=[0, 0, 0]  TranslationROffset=0  TranslationROffsetUnits=m  TranslationZOffset=0  TranslationZOffsetUnits=m  TranslationThetaOffset=0  TranslationThetaOffsetUnits=deg  RotationMethod=ArbitraryAxis  RotationAngleUnits=rad  RotationStandardAxis=+Z  RotationAngle=1.570796326794897  RotationArbitraryAxis=[-0, 1, 0]  FollAlignAxisA=+X  BaseAlignAxisA=+Y  FollAlignAxisB=+Y  BaseAlignAxisB=+Z  RotationSequenceAxes=FollowerAxes  RotationSequence=XYX  RotationSequenceAngles=[0 0 0]  RotationSequenceAnglesUnits=deg  RotationMatrix=[1 0 0; 0 1 0; 0 0 1]
  m1_OriginTransform : sm_lib/Frames and Transforms/Rigid Transform  TranslationMethod=Cartesian  TranslationStandardOffset=0  TranslationLengthUnit=m  TranslationStandardAxis=+Z  TranslationCartesianOffset=[0.0057356, 0.016065, -0.0165]  TranslationROffset=0  TranslationROffsetUnits=m  TranslationZOffset=0  TranslationZOffsetUnits=m  TranslationThetaOffset=0  TranslationThetaOffsetUnits=deg  RotationMethod=RotationSequence  RotationAngleUnits=deg  RotationStandardAxis=+Z  RotationAngle=0.0  RotationArbitraryAxis=[0 0 1]  FollAlignAxisA=+X  BaseAlignAxisA=+Y  FollAlignAxisB=+Y  BaseAlignAxisB=+Z  RotationSequenceAxes=BaseAxes  RotationSequence=XYZ  RotationSequenceAngles=[0, 0, 0]  RotationSequenceAnglesUnits=rad  RotationMatrix=[1 0 0; 0 1 0; 0 0 1]
  r1_AxisTransform : sm_lib/Frames and Transforms/Rigid Transform  TranslationMethod=Cartesian  TranslationStandardOffset=0  TranslationLengthUnit=m  TranslationStandardAxis=+Z  TranslationCartesianOffset=[0, 0, 0]  TranslationROffset=0  TranslationROffsetUnits=m  TranslationZOffset=0  TranslationZOffsetUnits=m  TranslationThetaOffset=0  TranslationThetaOffsetUnits=deg  RotationMethod=ArbitraryAxis  RotationAngleUnits=rad  RotationStandardAxis=+Z  RotationAngle=1.570796326794897  RotationArbitraryAxis=[-0, 1, 0]  FollAlignAxisA=+X  BaseAlignAxisA=+Y  FollAlignAxisB=+Y  BaseAlignAxisB=+Z  RotationSequenceAxes=FollowerAxes  RotationSequence=XYX  RotationSequenceAngles=[0 0 0]  RotationSequenceAnglesUnits=deg  RotationMatrix=[1 0 0; 0 1 0; 0 0 1]
  r1_OriginTransform : sm_lib/Frames and Transforms/Rigid Transform  TranslationMethod=Cartesian  TranslationStandardOffset=0  TranslationLengthUnit=m  TranslationStandardAxis=+Z  TranslationCartesianOffset=[-0.010616, 0.014956, -0.0165]  TranslationROffset=0  TranslationROffsetUnits=m  TranslationZOffset=0  TranslationZOffsetUnits=m  TranslationThetaOffset=0  TranslationThetaOffsetUnits=deg  RotationMethod=RotationSequence  RotationAngleUnits=deg  RotationStandardAxis=+Z  RotationAngle=0.0  RotationArbitraryAxis=[0 0 1]  FollAlignAxisA=+X  BaseAlignAxisA=+Y  FollAlignAxisB=+Y  BaseAlignAxisB=+Z  RotationSequenceAxes=BaseAxes  RotationSequence=XYZ  RotationSequenceAngles=[0, 0, 0.061087]  RotationSequenceAnglesUnits=rad  RotationMatrix=[1 0 0; 0 1 0; 0 0 1]
  t0_AxisTransform : sm_lib/Frames and Transforms/Rigid Transform  TranslationMethod=Cartesian  TranslationStandardOffset=0  TranslationLengthUnit=m  TranslationStandardAxis=+Z  TranslationCartesianOffset=[0, 0, 0]  TranslationROffset=0  TranslationROffsetUnits=m  TranslationZOffset=0  TranslationZOffsetUnits=m  TranslationThetaOffset=0  TranslationThetaOffsetUnits=deg  RotationMethod=ArbitraryAxis  RotationAngleUnits=rad  RotationStandardAxis=+Z  RotationAngle=1.570796326794897  RotationArbitraryAxis=[-0, -1, 0]  FollAlignAxisA=+X  BaseAlignAxisA=+Y  FollAlignAxisB=+Y  BaseAlignAxisB=+Z  RotationSequenceAxes=FollowerAxes  RotationSequence=XYX  RotationSequenceAngles=[0 0 0]  RotationSequenceAnglesUnits=deg  RotationMatrix=[1 0 0; 0 1 0; 0 0 1]
  t0_OriginTransform : sm_lib/Frames and Transforms/Rigid Transform  TranslationMethod=Cartesian  TranslationStandardOffset=0  TranslationLengthUnit=m  TranslationStandardAxis=+Z  TranslationCartesianOffset=[0.027262, -0.051234, 0.00015]  TranslationROffset=0  TranslationROffsetUnits=m  TranslationZOffset=0  TranslationZOffsetUnits=m  TranslationThetaOffset=0  TranslationThetaOffsetUnits=deg  RotationMethod=RotationSequence  RotationAngleUnits=deg  RotationStandardAxis=+Z  RotationAngle=0.0  RotationArbitraryAxis=[0 0 1]  FollAlignAxisA=+X  BaseAlignAxisA=+Y  FollAlignAxisB=+Y  BaseAlignAxisB=+Z  RotationSequenceAxes=BaseAxes  RotationSequence=XYZ  RotationSequenceAngles=[0, 0, -0.80285]  RotationSequenceAnglesUnits=rad  RotationMatrix=[1 0 0; 0 1 0; 0 0 1]
  F : PMIOPort  Side=Left
  t : PMIOPort  Port=2  Side=Right
  i : PMIOPort  Port=3  Side=Right
  m : PMIOPort  Port=4  Side=Right
  r : PMIOPort  Port=5  Side=Right
  l : PMIOPort  Port=6  Side=Right
  hand : PMIOPort  Port=7  Side=Right
  connections:
  Inertia/RConn1 -- InertiaOriginTransform/RConn1
  ReferenceFrame/RConn1 -- InertiaOriginTransform/LConn1 -- r1_OriginTransform/LConn1 -- t0_OriginTransform/LConn1 -- m1_OriginTransform/LConn1 -- l1_OriginTransform/LConn1 -- i1_OriginTransform/LConn1 -- VisualOriginTransform/LConn1 -- F/RConn1
  Visual/RConn1 -- hand/RConn1 -- VisualOriginTransform/RConn1
  i1_AxisTransform/RConn1 -- i/RConn1
  i1_AxisTransform/LConn1 -- i1_OriginTransform/RConn1
  l1_AxisTransform/RConn1 -- l/RConn1
  l1_AxisTransform/LConn1 -- l1_OriginTransform/RConn1
  m1_AxisTransform/RConn1 -- m/RConn1
  m1_AxisTransform/LConn1 -- m1_OriginTransform/RConn1
  r1_AxisTransform/RConn1 -- r/RConn1
  r1_AxisTransform/LConn1 -- r1_OriginTransform/RConn1
  t0_AxisTransform/RConn1 -- t/RConn1
  t0_AxisTransform/LConn1 -- t0_OriginTransform/RConn1

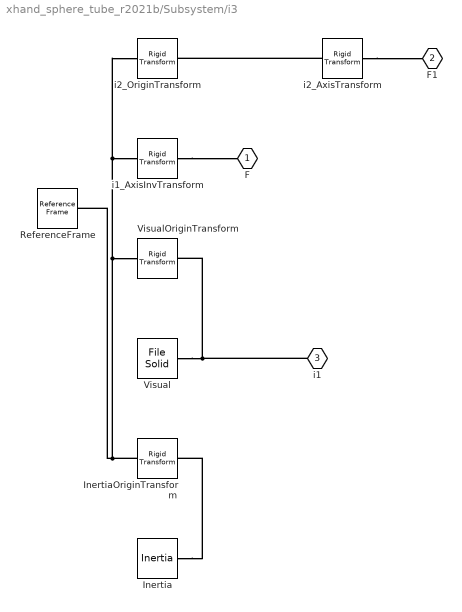
== system xhand_sphere_tube_r2021b/Subsystem/i3 ==
  Inertia : sm_lib/Body Elements/Inertia  InertiaType=Custom  Mass=0.00267269398389927  MassUnits=kg  CenterOfMass=[0, 0, 0]  CenterOfMassUnits=m  MomentsOfInertia=[3.76486307951961e-07, 8.47363849301882e-08, 3.8883243488867e-07]  MomentsOfInertiaUnits=kg*m^2  ProductsOfInertia=[8.10104158906665e-10, -1.31306405896085e-09, 1.82790945167911e-13]  ProductsOfInertiaUnits=kg*m^2  GraphicType=None  MarkerShape=Inertia  MarkerSize=20  GraphicVisPropType=SimpleVisualProperties  GraphicDiffuseColor=[0.5 0.5 0.5]  GraphicSpecularColor=[0.5 0.5 0.5 1.0]  GraphicAmbientColor=[0.15 0.15 0.15 1.0]  GraphicEmissiveColor=[0.0 0.0 0.0 1.0]  GraphicShininess=75  GraphicOpacity=1.0
  InertiaOriginTransform : sm_lib/Frames and Transforms/Rigid Transform  TranslationMethod=Cartesian  TranslationStandardOffset=0  TranslationLengthUnit=m  TranslationStandardAxis=+Z  TranslationCartesianOffset=[0.00199444388715324, 0.0173903557958, 9.448913471013511e-05]  TranslationROffset=0  TranslationROffsetUnits=m  TranslationZOffset=0  TranslationZOffsetUnits=m  TranslationThetaOffset=0  TranslationThetaOffsetUnits=deg  RotationMethod=RotationSequence  RotationAngleUnits=deg  RotationStandardAxis=+Z  RotationAngle=0.0  RotationArbitraryAxis=[0 0 1]  FollAlignAxisA=+X  BaseAlignAxisA=+Y  FollAlignAxisB=+Y  BaseAlignAxisB=+Z  RotationSequenceAxes=BaseAxes  RotationSequence=XYZ  RotationSequenceAngles=[0, 0, 0]  RotationSequenceAnglesUnits=rad  RotationMatrix=[1 0 0; 0 1 0; 0 0 1]
  ReferenceFrame : sm_lib/Frames and Transforms/Reference Frame
  Visual : sm_lib/Body Elements/File Solid  ExtGeomFileName=xhand/meshes/i1.STL  UnitType=Custom  ExtGeomFileUnits=m  StepReaderType=HEX  ExportConvexHullGeometry=off  InertiaType=Custom  Mass=0  MassUnits=kg  CenterOfMass=[0, 0, 0]  CenterOfMassUnits=m  MomentsOfInertia=[0, 0, 0]  MomentsOfInertiaUnits=kg*m^2  ProductsOfInertia=[0, 0, 0]  ProductsOfInertiaUnits=kg*m^2  BasedOnType=DensityFromFile  Density=1000  DensityUnits=kg/m^3  DoExposeReferenceFrame=on  SerializedFrames=<Frames/>  GraphicType=FromGeometry  MarkerShape=Sphere  MarkerSize=10  GraphicVisPropType=SimpleVisualProperties  GraphicDiffuseColor=[1, 1, 1]  GraphicSpecularColor=[0.5 0.5 0.5 1.0]  GraphicAmbientColor=[0.15 0.15 0.15 1.0]  GraphicEmissiveColor=[0.0 0.0 0.0 1.0]  GraphicShininess=75  GraphicOpacity=1
  VisualOriginTransform : sm_lib/Frames and Transforms/Rigid Transform  TranslationMethod=Cartesian  TranslationStandardOffset=0  TranslationLengthUnit=m  TranslationStandardAxis=+Z  TranslationCartesianOffset=[0, 0, 0]  TranslationROffset=0  TranslationROffsetUnits=m  TranslationZOffset=0  TranslationZOffsetUnits=m  TranslationThetaOffset=0  TranslationThetaOffsetUnits=deg  RotationMethod=RotationSequence  RotationAngleUnits=deg  RotationStandardAxis=+Z  RotationAngle=0.0  RotationArbitraryAxis=[0 0 1]  FollAlignAxisA=+X  BaseAlignAxisA=+Y  FollAlignAxisB=+Y  BaseAlignAxisB=+Z  RotationSequenceAxes=BaseAxes  RotationSequence=XYZ  RotationSequenceAngles=[0, 0, 0]  RotationSequenceAnglesUnits=rad  RotationMatrix=[1 0 0; 0 1 0; 0 0 1]
  i1_AxisInvTransform : sm_lib/Frames and Transforms/Rigid Transform  TranslationMethod=Cartesian  TranslationStandardOffset=0  TranslationLengthUnit=m  TranslationStandardAxis=+Z  TranslationCartesianOffset=[0, 0, 0]  TranslationROffset=0  TranslationROffsetUnits=m  TranslationZOffset=0  TranslationZOffsetUnits=m  TranslationThetaOffset=0  TranslationThetaOffsetUnits=deg  RotationMethod=ArbitraryAxis  RotationAngleUnits=rad  RotationStandardAxis=+Z  RotationAngle=1.570796326794897  RotationArbitraryAxis=[-0, 1, 0]  FollAlignAxisA=+X  BaseAlignAxisA=+Y  FollAlignAxisB=+Y  BaseAlignAxisB=+Z  RotationSequenceAxes=FollowerAxes  RotationSequence=XYX  RotationSequenceAngles=[0 0 0]  RotationSequenceAnglesUnits=deg  RotationMatrix=[1 0 0; 0 1 0; 0 0 1]
  i2_AxisTransform : sm_lib/Frames and Transforms/Rigid Transform  TranslationMethod=Cartesian  TranslationStandardOffset=0  TranslationLengthUnit=m  TranslationStandardAxis=+Z  TranslationCartesianOffset=[0, 0, 0]  TranslationROffset=0  TranslationROffsetUnits=m  TranslationZOffset=0  TranslationZOffsetUnits=m  TranslationThetaOffset=0  TranslationThetaOffsetUnits=deg  RotationMethod=ArbitraryAxis  RotationAngleUnits=rad  RotationStandardAxis=+Z  RotationAngle=1.570796326794897  RotationArbitraryAxis=[-0, -1, 0]  FollAlignAxisA=+X  BaseAlignAxisA=+Y  FollAlignAxisB=+Y  BaseAlignAxisB=+Z  RotationSequenceAxes=FollowerAxes  RotationSequence=XYX  RotationSequenceAngles=[0 0 0]  RotationSequenceAnglesUnits=deg  RotationMatrix=[1 0 0; 0 1 0; 0 0 1]
  i2_OriginTransform : sm_lib/Frames and Transforms/Rigid Transform  TranslationMethod=Cartesian  TranslationStandardOffset=0  TranslationLengthUnit=m  TranslationStandardAxis=+Z  TranslationCartesianOffset=[0.004, 0.03777, 0]  TranslationROffset=0  TranslationROffsetUnits=m  TranslationZOffset=0  TranslationZOffsetUnits=m  TranslationThetaOffset=0  TranslationThetaOffsetUnits=deg  RotationMethod=RotationSequence  RotationAngleUnits=deg  RotationStandardAxis=+Z  RotationAngle=0.0  RotationArbitraryAxis=[0 0 1]  FollAlignAxisA=+X  BaseAlignAxisA=+Y  FollAlignAxisB=+Y  BaseAlignAxisB=+Z  RotationSequenceAxes=BaseAxes  RotationSequence=XYZ  RotationSequenceAngles=[0.10471975511966, 0, 0]  RotationSequenceAnglesUnits=rad  RotationMatrix=[1 0 0; 0 1 0; 0 0 1]
  F : PMIOPort  Side=Left
  F1 : PMIOPort  Port=2  Side=Right
  i1 : PMIOPort  Port=3  Side=Left
  connections:
  Inertia/RConn1 -- InertiaOriginTransform/RConn1
  ReferenceFrame/RConn1 -- InertiaOriginTransform/LConn1 -- i1_AxisInvTransform/LConn1 -- i2_OriginTransform/LConn1 -- VisualOriginTransform/LConn1
  Visual/RConn1 -- i1/RConn1 -- VisualOriginTransform/RConn1
  i1_AxisInvTransform/RConn1 -- F/RConn1
  i2_AxisTransform/RConn1 -- F1/RConn1
  i2_AxisTransform/LConn1 -- i2_OriginTransform/RConn1
